simulink model "LinearModelWithObserver"  (R2022a)
settings: Solver=FixedStepAuto  StartTime=0.0  StopTime=inf  FixedStep=0.01  MaxStep=1e-3  MinStep=1e-5  RelTol=1e-3  EnableMultiTasking=on
values from neighbouring files (symbols this model uses):
  A = A_lin    [parameter_values.m]
  B = B_lin    [parameter_values.m]
  C1 = [1 0 0 0]    [parameter_values.m]
  C_obs = [1 0 0 0; 0 0 1 0]    [parameter_values.m]
  K_lmi = calc_LMI_Controller(A,B,0.5)    [parameter_values.m]
  L = inv(P_sol)*N_sol    [calc_LMI_Observer.m]    (also in parameter_values.m = calc_LMI_Observer(A,C_obs,10))
  x0 = [deg2rad(0.1); 0; 0; 0]    [parameter_values.m]
  x_hat_0 = [0 0 0 0]    [parameter_values.m]
libraries: svdutilitieslib x1, mbedblockslib x1
settings Model: ExtModeTrigDuration=10  Creator=schulte  LastModifiedBy=adlipke
settings SolverCC: AlgebraicLoopSolver=TrustRegion
settings DataIOCC: ReturnWorkspaceOutputs=off
settings OptimizationCC: EnhancedBackFolding=on  PassReuseOutputArgsAs=Individual arguments  ZeroExternalMemoryAtStartup=off  ZeroInternalMemoryAtStartup=off  MaxStackSize=64  OptimizeBlockOrder=speed  DifferentSizesBufferReuse=on  OptimizationCustomize=off  EfficientTunableParamExpr=on
settings DebuggingCC: ParameterTunabilityLossMsg=error  UnconnectedInputMsg=warning  UnconnectedOutputMsg=warning  UnconnectedLineMsg=warning  SFUnexpectedBacktrackingDiag=warning  SFNoUnconditionalDefaultTransitionDiag=warning  SFMachineParentedDataDiag=warning  ArithmeticOperatorsInVariantConditions=warning
settings HardwareCC: ProdBitPerPointer=32  ProdBitPerSizeT=32  ProdBitPerPtrDiffT=32  ProdLargestAtomicInteger=Long  ProdLargestAtomicFloat=Double  ProdWordSize=32  ProdLongLongMode=on  ProdHWDeviceType=ARM Compatible->ARM Cortex
settings SFSimCC: SimUseLocalCustomCode=off  MATLABDynamicMemAlloc=off  CustomCodeUndefinedFunction=UseInterfaceOnly
settings RTWCC: SystemTargetFile=ert.tlc  HardwareBoard=STM32 Nucleo L476RG  TemplateMakefile=ert_default_tmf  RTWUseLocalCustomCode=off  Toolchain=GNU Tools for ARM Embedded Processors
settings CodeAppCC: ForceParamTrailComments=on  IgnoreCustomStorageClasses=off  OperatorAnnotations=on  SimulinkDataObjDesc=on  SFDataObjDesc=on  InsertBlockDesc=on
settings ERTTargetCC: SupportContinuousTime=on  ExtModeTransport=3  ExtModeStaticAlloc=on  ExtModeStaticAllocSize=2000  ExtModeMexFile=ext_xcp  ExtModeIntrfLevel=Level2 - Open
settings ConfigComp: CovMetricSettings=dw  CovSaveCumulativeToWorkspaceVar=on  CovSaveSingleToWorkspaceVar=on  CovExternalEMLEnable=off

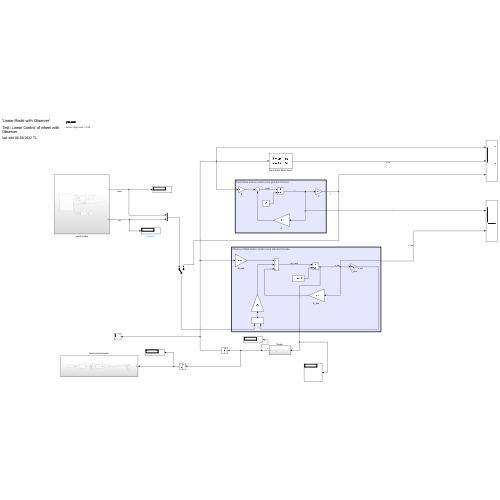
[thumbnail: Simulink's stored preview of the top-level diagram]
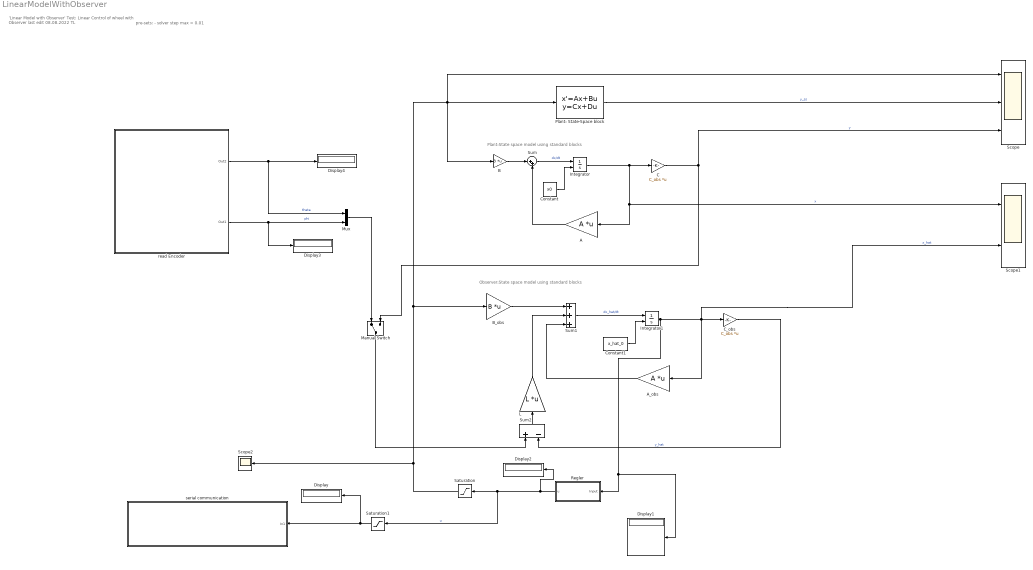
== system LinearModelWithObserver ==
  note: Observer:State space model using standard blocks
  note: Plant:State space model using standard blocks
  note: pre-sets:
      |
      | - solver step max = 0.01
  note: 'Linear Model with Observer'
      |
      | Test: Linear Control of wheel with Observer
      |
      | last edit 08.08.2022 TL
  A : Gain  Gain=A  Multiplication=Matrix(K*u)
  A_obs : Gain  Gain=A  Multiplication=Matrix(K*u)
  B : Gain  Gain=B  Multiplication=Matrix(K*u)
  B_obs : Gain  Gain=B  Multiplication=Matrix(K*u)
  C : Gain  Gain=C_obs  Multiplication=Matrix(K*u)
  C_obs : Gain  Gain=C_obs  Multiplication=Matrix(K*u)
  Constant : Constant  Value=x0
  Constant1 : Constant  Value=x_hat_0
  Display{,1..4} (5 alike) : Display
  Integrator : Integrator  InitialConditionSource=external  InitialCondition=x0
  Integrator1 : Integrator  InitialConditionSource=external  InitialCondition=x0
  L : Gain  Gain=L  Multiplication=Matrix(K*u)
  Manual Switch : ManualSwitch
  Mux : Mux  Inputs=2
  Plant: State-Space block : StateSpace  A=A  B=B  C=C1  D=0  InitialCondition=x0
  Regler : Subsystem
  Saturation : Saturate  UpperLimit=10  LowerLimit=-10
  Saturation1 : Saturate  UpperLimit=12  LowerLimit=-12
  Scope : Scope  NumInputPorts=3
  Scope1 : Scope  NumInputPorts=2
  Scope2 : Scope
  Sum : Sum  Inputs=|++
  Sum1 : Sum  Inputs=+++
  Sum2 : Sum  Inputs=+-
  read Encoder : Subsystem
  serial communication : Subsystem
  wires:
  Regler/1(u) -> Display2/1, Saturation1/1, Saturation/1  "u"
  Plant: State-Space block/1 -> Scope/2  "y_ss"
  A/1 -> Sum/2
  B/1 -> Sum/1
  Sum/1 -> Integrator/1  "dx/dt"
  Integrator/1 -> C/1, A/1, Scope1/1  "x"
  C/1 -> Manual Switch/2, Scope/3  "y"
  Constant/1 -> Integrator/2
  A_obs/1 -> Sum1/3
  Sum2/1 -> L/1
  L/1 -> Sum1/2
  Sum1/1 -> Integrator1/1  "dx_hat/dt"
  C_obs/1 -> Sum2/2  "y_hat"
  Integrator1/1 -> Display1/1, Regler/1(Input), Scope1/2, C_obs/1, A_obs/1  "x_hat"
  B_obs/1 -> Sum1/1
  Constant1/1 -> Integrator1/2
  Saturation/1 -> Scope2/1, Plant: State-Space block/1, Scope/1, B/1, B_obs/1
  Mux/1 -> Manual Switch/1
  Manual Switch/1 -> Sum2/1
  Saturation1/1 -> Display/1, serial communication/1(In1)
  read Encoder/2(Out1) -> Display3/1, Mux/2  "phi"
  read Encoder/1(Out2) -> Mux/1, Display4/1  "theta"

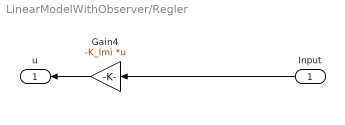
== system LinearModelWithObserver/Regler ==
  Input : Inport
  Gain4 : Gain  Gain=-K_lmi  Multiplication=Matrix(K*u)
  u : Outport
  wires:
  Gain4/1 -> u/1
  Input/1 -> Gain4/1

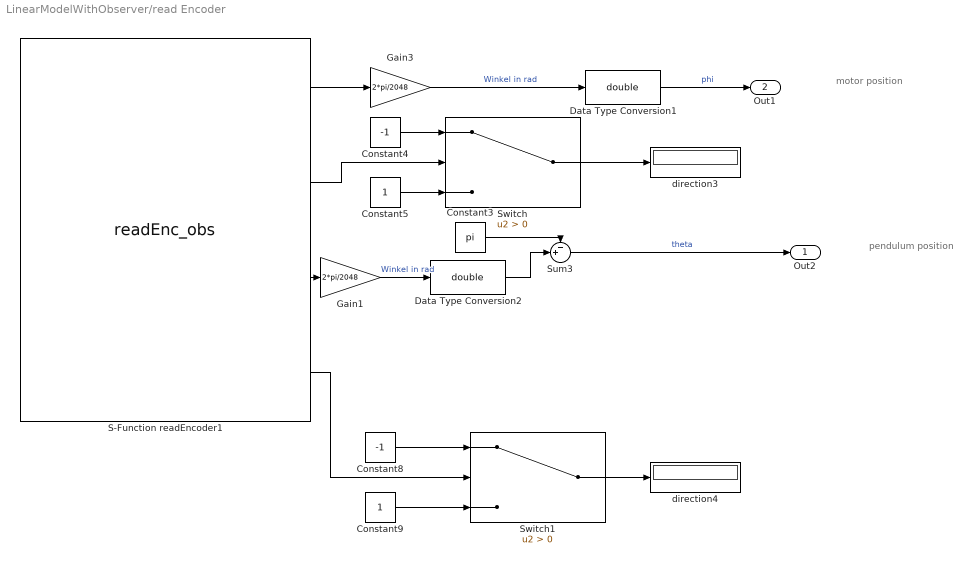
== system LinearModelWithObserver/read Encoder ==
  note: motor position
  note: pendulum position
  Constant3 : Constant  Value=pi
  Constant4 : Constant  Value=-1
  Constant5 : Constant
  Constant8 : Constant  Value=-1
  Constant9 : Constant
  Data Type Conversion1 : DataTypeConversion  OutDataTypeStr=double  SaturateOnIntegerOverflow=off  RndMeth=Floor
  Data Type Conversion2 : DataTypeConversion  OutDataTypeStr=double  SaturateOnIntegerOverflow=off  RndMeth=Floor
  Gain1 : Gain  Gain=2*pi/2048
  Gain3 : Gain  Gain=2*pi/2048
  S-Function readEncoder1 : S-Function  FunctionName=readEnc_obs  SFunctionModules=readEnc_obs_wrapper  SFunctionDeploymentMode=off  EnableBusSupport=off  mask(S-Function Builder){}
      mask help: Simulink:masks:SFunctionBuilder_MD
      mask init:
      | val = [[.9  0.75 0.75 1 1 .9 .9 1]',[1 1 0.75 0.75 .9 .9 1 .9]'];try , sys = get_param(gcb,'SfunBuilderFcnName');if isempty(sys), sys = get_param(gcb,'FunctionName'); end,catch, sys = get_param(gcb,'FunctionName'); end
      settings: CopyFcn=set_param(gcbh,'LinkStatus','none')  OpenFcn=sfunctionwizard(gcbh)
      mask Display:
      | plot(val(:,1),val(:,2))
      | disp(sys)
      | port_label('output',1,'tim2_cnt')
      | port_label('output',2,'tim2_dir')
      | port_label('output',3,'tim3_cnt')
      | port_label('output',4,'tim3_dir')
  Sum3 : Sum  Inputs=-+|
  Switch : Switch  Criteria=u2 > Threshold  SaturateOnIntegerOverflow=off  InputSameDT=off
  Switch1 : Switch  Criteria=u2 > Threshold  SaturateOnIntegerOverflow=off  InputSameDT=off
  direction3 : Display
  direction4 : Display
  Out2 : Outport
  Out1 : Outport  Port=2
  wires:
  Constant4/1 -> Switch/1
  Constant5/1 -> Switch/3
  S-Function readEncoder1/1 -> Gain3/1
  S-Function readEncoder1/4 -> Switch1/2
  Switch1/1 -> direction4/1
  S-Function readEncoder1/3 -> Gain1/1
  Constant8/1 -> Switch1/1
  Constant9/1 -> Switch1/3
  Gain3/1 -> Data Type Conversion1/1  "Winkel in rad"
  Data Type Conversion2/1 -> Sum3/2
  Switch/1 -> direction3/1
  Gain1/1 -> Data Type Conversion2/1  "Winkel in rad"
  Constant3/1 -> Sum3/1
  S-Function readEncoder1/2 -> Switch/2
  Sum3/1 -> Out2/1  "theta"
  Data Type Conversion1/1 -> Out1/1  "phi"

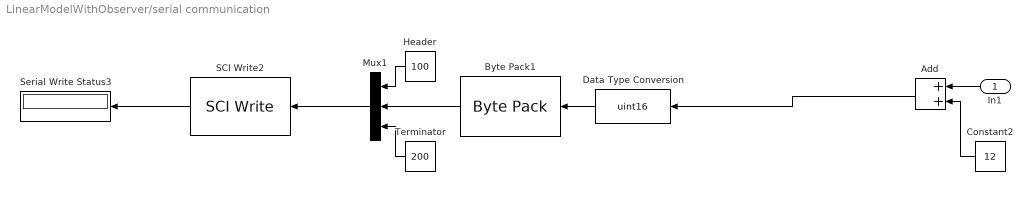
== system LinearModelWithObserver/serial communication ==
  In1 : Inport
  Add : Sum  AccumDataTypeStr=uint16  OutDataTypeStr=uint16
  Byte Pack1 : svdutilitieslib/Byte Pack  maskPackedDataType=uint8  datatypes={'uint16'}  byteAlign=1  blockPlatform=arduinoert
      settings: SourceProductBaseCode=ANDROID,ARDUINO,ML_ARDUINO,ECCORTEXA,ECCORTEXR,SC_BEAGLEBONE_BLUE,EC_FREEDOM_BOARD,EC_FRDM_K64F,INTEL_BLOCKSET,MICROBIT,NUCLEO,NVIDIA,PX4AUTOPILOTS,RASPPIIO,STMICRODIS,TIC2000,XILINX_BLOCKSET
  Constant2 : Constant  Value=12  OutDataTypeStr=single
  Data Type Conversion : DataTypeConversion  OutDataTypeStr=uint16  SaturateOnIntegerOverflow=off  RndMeth=Floor
  Header : Constant  Value=100  OutDataTypeStr=uint8  SampleTime=0.01
  Mux1 : Mux  Inputs=3
  SCI Write2 : mbedblockslib/SCI Write  SCIModule=1  Baudrate=uint32(9600)  Parity=None  StopBits=1  HardwareFlowControl=None  ByteOrder=LittleEndian  OutputStatus=on
      settings: SourceProductBaseCode=MICROBIT,NUCLEO,STMICRODIS
  Serial Write Status3 : Display
  Terminator : Constant  Value=200  OutDataTypeStr=uint8  SampleTime=0.01
  wires:
  Mux1/1 -> SCI Write2/1
  Terminator/1 -> Mux1/3
  Byte Pack1/1 -> Mux1/2
  Add/1 -> Data Type Conversion/1
  Data Type Conversion/1 -> Byte Pack1/1
  SCI Write2/1 -> Serial Write Status3/1
  Header/1 -> Mux1/1
  Constant2/1 -> Add/2
  In1/1 -> Add/1
